simulink model "test_udp"  (R2021b)
settings: Solver=FixedStepAuto  StartTime=0.0  StopTime=inf  FixedStep=0.01  RelTol=1e-3
libraries: dspnetwork x3
settings Model: Creator=takeh  LastModifiedBy=takeh

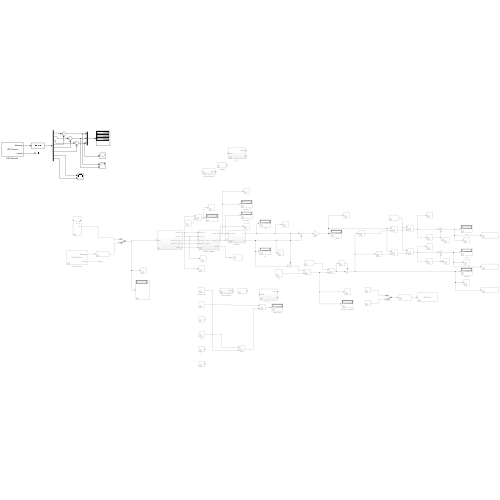
[thumbnail: Simulink's stored preview of the top-level diagram]
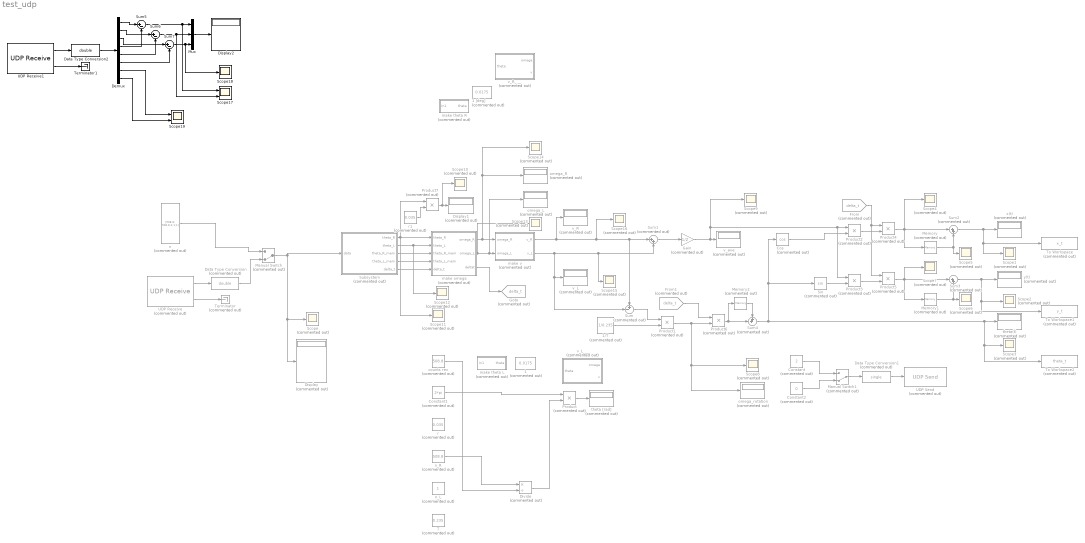
== system test_udp ==
  1 : Constant  Commented=on  Value=0.0175
  1 [deg] : Constant  Commented=on  Value=0.0175
  1/T : Constant  Commented=on  Value=1/0.235
  Constant : Constant  Commented=on  Value=2
  Constant1 : Constant  Commented=on  Value=2*pi
  Constant2 : Constant  Commented=on  Value=0
  Cos : Trigonometry  Commented=on  Operator=cos
  Data Type Conversion : DataTypeConversion  Commented=on  OutDataTypeStr=double
  Data Type Conversion1 : DataTypeConversion  Commented=on  OutDataTypeStr=single
  Data Type Conversion2 : DataTypeConversion  OutDataTypeStr=double
  Demux : Demux  Outputs=8
  Display : Display  Commented=on
  Display1 : Display  Commented=on
  Display2 : Display
  Divide : Product  Commented=on  Inputs=*/
  From : From  Commented=on  GotoTag=delta_t  TagVisibility=global
  From1 : From  Commented=on  GotoTag=delta_t  TagVisibility=global
  Gain : Gain  Commented=on  Gain=1/2
  Goto : Goto  Commented=on  GotoTag=delta_t  TagVisibility=global
  Manual Switch : ManualSwitch  Commented=on  CurrentSetting=0
  Manual Switch1 : ManualSwitch  Commented=on  CurrentSetting=0
  Memory : Memory  Commented=on
  Memory1 : Memory  Commented=on
  Memory2 : Memory  Commented=on
  Mux : Mux  Inputs=3
  Product{,1..7} (8 alike) : Product  Commented=on
  Scope{,1..16} (17 alike) : Scope  Commented=on
  Scope17 : Scope  NumInputPorts=2
  Scope18 : Scope
  Scope19 : Scope  NumInputPorts=2
  Sin : Trigonometry  Commented=on
  Subsystem : Subsystem  Commented=on
  Sum : Sum  Commented=on  Inputs=+-|
  Sum1 : Sum  Commented=on  Inputs=|++
  Sum2 : Sum  Commented=on  Inputs=|++
  Sum3 : Sum  Commented=on  Inputs=|++
  Sum4 : Sum  Commented=on  Inputs=++|
  Sum5 : Sum  Inputs=|+-
  Sum6 : Sum  Inputs=|+-
  Sum7 : Sum  Inputs=|+-
  T : Constant  Commented=on  Value=0.235
  Terminator : Terminator  Commented=on
  Terminator1 : Terminator
  To Workspace : ToWorkspace  Commented=on  VariableName=x_t  SaveFormat=Timeseries  SampleTime=-1
  To Workspace1 : ToWorkspace  Commented=on  VariableName=y_t  SaveFormat=Timeseries  SampleTime=-1
  To Workspace2 : ToWorkspace  Commented=on  VariableName=theta_t  SaveFormat=Timeseries  SampleTime=-1
  UDP Receive : dspnetwork/UDP Receive  Commented=on  localURL='0.0.0.0'  localPort=51000  remoteURL='127.0.0.1'  remotePort=-1  recvBufferSize=20  dims=5  signalDatatype=single  isComplex=off  isVarSize=off  showBlockingTime=off  blockingTime=0  sampletime=-1  blockPlatform=[]
  UDP Receive1 : dspnetwork/UDP Receive  localURL='0.0.0.0'  localPort=51000  remoteURL='127.0.0.1'  remotePort=-1  recvBufferSize=32  dims=8  signalDatatype=single  isComplex=off  isVarSize=off  showBlockingTime=off  blockingTime=0  sampletime=-1  blockPlatform=[]
  UDP Send : dspnetwork/UDP Send  Commented=on  remoteURL='127.0.0.1'  remotePort=52000  localURL='0.0.0.0'  localPortSource=Automatically determine  localPort=-1  sendBufferSize=8192  sampletime=-1  blockPlatform=[]  separateLengthPort=0
  counts rev : Constant  Commented=on  Value=508.8
  make omega : Subsystem  Commented=on
  make theta L : Subsystem  Commented=on
  make theta R : Subsystem  Commented=on
  make v : Subsystem  Commented=on
  n : Constant  Commented=on  Value=[508.8; 508.8;1;1;1]  VectorParams1D=off
  n_L : Constant  Commented=on
  n_R : Constant  Commented=on  Value=508.8
  omega_L : Display  Commented=on
  omega_R : Display  Commented=on
  omega_rotation : Display  Commented=on
  r : Constant  Commented=on  Value=0.035
  r1 : Constant  Commented=on  Value=0.035
  theta [rad] : Display  Commented=on
  theta(t) : Display  Commented=on
  v_L : Display  Commented=on
  v_L___ : Subsystem  Commented=on
  v_R : Display  Commented=on
  v_R____ : Subsystem  Commented=on
  v_ave : Display  Commented=on
  x(t) : Display  Commented=on
  y(t) : Display  Commented=on
  wires:
  UDP Receive/1 -> Data Type Conversion/1
  UDP Receive/2 -> Terminator/1
  Data Type Conversion/1 -> Manual Switch/2
  n/1 -> Manual Switch/1
  counts rev/1 -> Divide/2
  n_R/1 -> Divide/1
  Divide/1 -> Product/2
  Constant1/1 -> Product/1
  Product/1 -> theta [rad]/1
  1/T/1 -> Product1/2
  Sum/1 -> Product1/1
  Sum1/1 -> Gain/1
  Gain/1 -> Scope9/1, Product3/1, Product2/1, v_ave/1
  Sum4/1 -> To Workspace2/1, Scope3/1, theta(t)/1, Cos/1, Sin/1
  Cos/1 -> Product2/2
  Sin/1 -> Product3/2
  Sum3/1 -> y(t)/1, To Workspace1/1, Scope2/1
  make omega/1(omega_R) -> Scope14/1, omega_R/1, make v/1(omega_R)
  make v/1(v_R) -> Scope16/1, Sum1/1, Sum/1, v_R/1
  make v/2(v_L) -> Sum/2, v_L/1, Sum1/2, Scope15/1
  Constant/1 -> Manual Switch1/1
  Constant2/1 -> Manual Switch1/2
  Manual Switch1/1 -> Data Type Conversion1/1
  Data Type Conversion1/1 -> UDP Send/1
  Product2/1 -> Product4/2
  From/1 -> Product4/1, Product5/1
  Product3/1 -> Product5/2
  Sum2/1 -> x(t)/1, Scope1/1, To Workspace/1
  Memory/1 -> Sum2/2, Scope5/1
  Product5/1 -> Scope7/1, Memory1/1, Sum3/1
  Memory1/1 -> Scope6/1, Sum3/2
  Manual Switch/1 -> Subsystem/1(data), Scope/1, Display/1
  Subsystem/5(delta_t) -> make omega/5(delta_t)
  Subsystem/2(theta_L) -> Scope12/1, make omega/2(theta_L)
  Subsystem/3(theta_R_mem) -> make omega/3(theta_R_mem)
  Subsystem/4(theta_L_mem) -> make omega/4(theta_L_mem)
  make omega/3(deltat) -> Goto/1
  From1/1 -> Product6/1
  Product1/1 -> Product6/2, Scope8/1, omega_rotation/1
  Product6/1 -> Memory2/1, Sum4/2
  Memory2/1 -> Sum4/1
  Product4/1 -> Scope4/1, Sum2/1, Memory/1
  r1/1 -> Product7/2
  Product7/1 -> Scope10/1, Display1/1
  Subsystem/1(theta_R) -> Scope11/1, Product7/1, make omega/1(theta_R)
  make omega/2(omega_L) -> Scope13/1, make v/2(omega_L), omega_L/1
  UDP Receive1/1 -> Data Type Conversion2/1
  UDP Receive1/2 -> Terminator1/1
  Data Type Conversion2/1 -> Demux/1
  Demux/1 -> Sum5/1
  Demux/4 -> Sum5/2
  Demux/2 -> Sum6/1
  Demux/5 -> Sum6/2
  Demux/3 -> Sum7/1
  Demux/6 -> Sum7/2
  Sum6/1 -> Scope17/2, Mux/2
  Sum7/1 -> Scope18/1, Mux/3
  Sum5/1 -> Scope17/1, Mux/1
  Mux/1 -> Display2/1
  Demux/7 -> Scope19/1
  Demux/8 -> Scope19/2

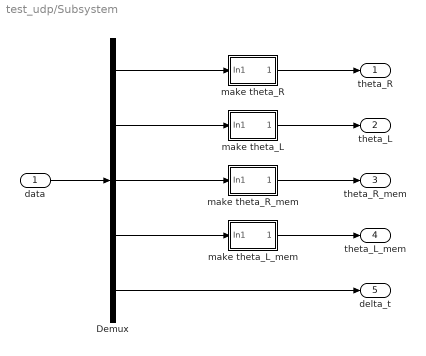
== system test_udp/Subsystem ==
  data : Inport
  Demux : Demux  Outputs=5
  make theta_L : Subsystem
  make theta_L_mem : Subsystem
  make theta_R : Subsystem
  make theta_R_mem : Subsystem
  theta_R : Outport
  theta_L : Outport  Port=2
  theta_R_mem : Outport  Port=3
  theta_L_mem : Outport  Port=4
  delta_t : Outport  Port=5
  wires:
  Demux/1 -> make theta_R/1(In1)
  make theta_R_mem/1(Out1) -> theta_R_mem/1
  Demux/3 -> make theta_R_mem/1(In1)
  make theta_L_mem/1(Out1) -> theta_L_mem/1
  Demux/2 -> make theta_L/1(In1)
  make theta_R/1(Out1) -> theta_R/1
  Demux/4 -> make theta_L_mem/1(In1)
  Demux/5 -> delta_t/1
  data/1 -> Demux/1
  make theta_L/1(Out1) -> theta_L/1

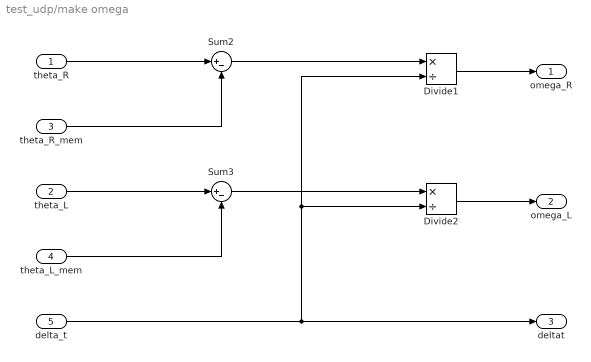
== system test_udp/make omega ==
  theta_R : Inport
  theta_L : Inport  Port=2
  theta_R_mem : Inport  Port=3
  theta_L_mem : Inport  Port=4
  delta_t : Inport  Port=5
  Divide1 : Product  Inputs=*/
  Divide2 : Product  Inputs=*/
  Sum2 : Sum  Inputs=|+-
  Sum3 : Sum  Inputs=|+-
  omega_R : Outport
  omega_L : Outport  Port=2
  deltat : Outport  Port=3
  wires:
  Sum2/1 -> Divide1/1
  Divide1/1 -> omega_R/1
  Sum3/1 -> Divide2/1
  Divide2/1 -> omega_L/1
  theta_R/1 -> Sum2/1
  theta_R_mem/1 -> Sum2/2
  theta_L/1 -> Sum3/1
  theta_L_mem/1 -> Sum3/2
  delta_t/1 -> deltat/1, Divide1/2, Divide2/2

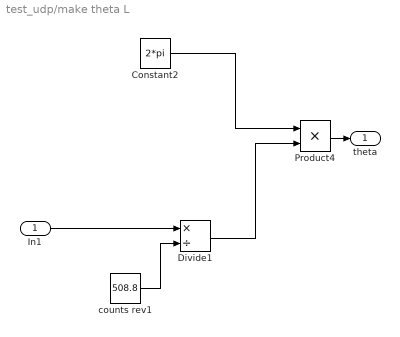
== system test_udp/make theta L ==
  In1 : Inport
  Constant2 : Constant  Value=2*pi
  Divide1 : Product  Inputs=*/
  Product4 : Product
  counts rev1 : Constant  Value=508.8
  theta : Outport
  wires:
  counts rev1/1 -> Divide1/2
  Constant2/1 -> Product4/1
  Divide1/1 -> Product4/2
  Product4/1 -> theta/1
  In1/1 -> Divide1/1

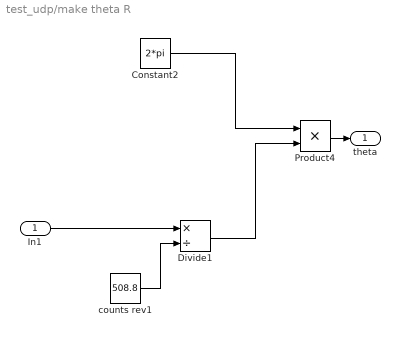
== system test_udp/make theta R ==
  In1 : Inport
  Constant2 : Constant  Value=2*pi
  Divide1 : Product  Inputs=*/
  Product4 : Product
  counts rev1 : Constant  Value=508.8
  theta : Outport
  wires:
  counts rev1/1 -> Divide1/2
  Constant2/1 -> Product4/1
  Divide1/1 -> Product4/2
  Product4/1 -> theta/1
  In1/1 -> Divide1/1

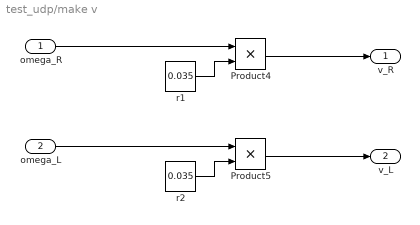
== system test_udp/make v ==
  omega_R : Inport
  omega_L : Inport  Port=2
  Product4 : Product
  Product5 : Product
  r1 : Constant  Value=0.035
  r2 : Constant  Value=0.035
  v_R : Outport
  v_L : Outport  Port=2
  wires:
  r2/1 -> Product5/2
  Product5/1 -> v_L/1
  Product4/1 -> v_R/1
  r1/1 -> Product4/2
  omega_R/1 -> Product4/1
  omega_L/1 -> Product5/1

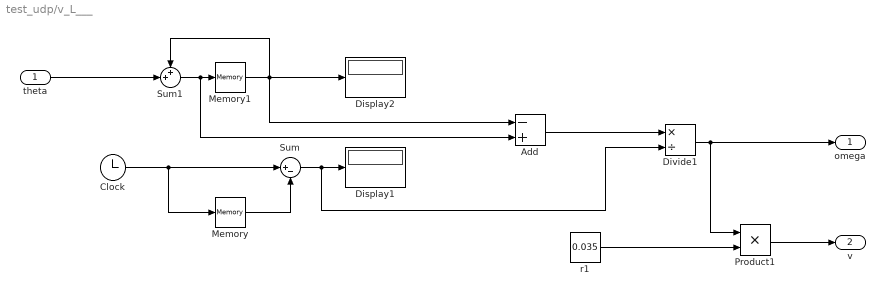
== system test_udp/v_L___ ==
  theta : Inport
  Add : Sum  Inputs=-+
  Clock : Clock
  Display1 : Display
  Display2 : Display
  Divide1 : Product  Inputs=*/
  Memory : Memory  InitialCondition=1
  Memory1 : Memory  InitialCondition=1
  Product1 : Product
  Sum : Sum  Inputs=|+-
  Sum1 : Sum  Inputs=++|
  r1 : Constant  Value=0.035
  omega : Outport
  v : Outport  Port=2
  wires:
  Memory1/1 -> Add/1, Display2/1, Sum1/1
  r1/1 -> Product1/2
  Sum1/1 -> Add/2, Memory1/1
  Sum/1 -> Divide1/2, Display1/1
  Memory/1 -> Sum/2
  Clock/1 -> Memory/1, Sum/1
  Add/1 -> Divide1/1
  Divide1/1 -> omega/1, Product1/1
  theta/1 -> Sum1/2
  Product1/1 -> v/1

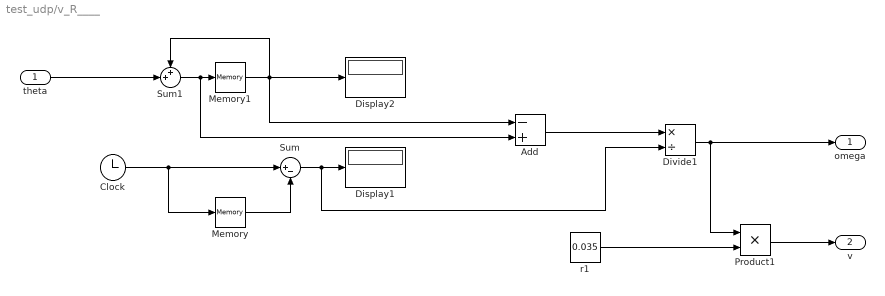
== system test_udp/v_R____ ==
  theta : Inport
  Add : Sum  Inputs=-+
  Clock : Clock
  Display1 : Display
  Display2 : Display
  Divide1 : Product  Inputs=*/
  Memory : Memory  InitialCondition=1
  Memory1 : Memory  InitialCondition=1
  Product1 : Product
  Sum : Sum  Inputs=|+-
  Sum1 : Sum  Inputs=++|
  r1 : Constant  Value=0.035
  omega : Outport
  v : Outport  Port=2
  wires:
  Memory1/1 -> Add/1, Display2/1, Sum1/1
  r1/1 -> Product1/2
  Sum1/1 -> Add/2, Memory1/1
  Sum/1 -> Divide1/2, Display1/1
  Memory/1 -> Sum/2
  Clock/1 -> Memory/1, Sum/1
  Add/1 -> Divide1/1
  Divide1/1 -> omega/1, Product1/1
  theta/1 -> Sum1/2
  Product1/1 -> v/1

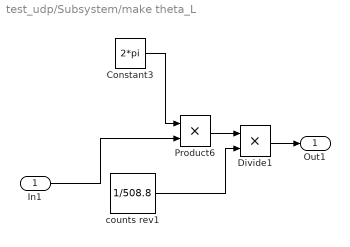
== system test_udp/Subsystem/make theta_L ==
  In1 : Inport
  Constant3 : Constant  Value=2*pi
  Divide1 : Product
  Product6 : Product
  counts rev1 : Constant  Value=1/508.8
  Out1 : Outport
  wires:
  Divide1/1 -> Out1/1
  In1/1 -> Product6/2
  counts rev1/1 -> Divide1/2
  Constant3/1 -> Product6/1
  Product6/1 -> Divide1/1

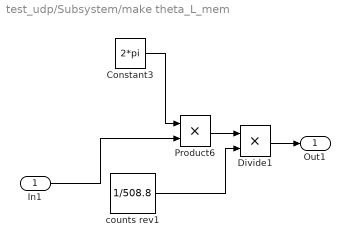
== system test_udp/Subsystem/make theta_L_mem ==
  In1 : Inport
  Constant3 : Constant  Value=2*pi
  Divide1 : Product
  Product6 : Product
  counts rev1 : Constant  Value=1/508.8
  Out1 : Outport
  wires:
  Divide1/1 -> Out1/1
  In1/1 -> Product6/2
  counts rev1/1 -> Divide1/2
  Constant3/1 -> Product6/1
  Product6/1 -> Divide1/1

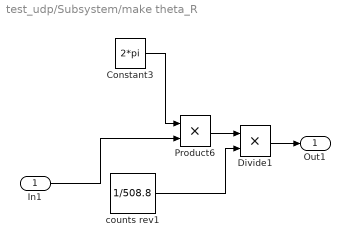
== system test_udp/Subsystem/make theta_R ==
  In1 : Inport
  Constant3 : Constant  Value=2*pi
  Divide1 : Product
  Product6 : Product
  counts rev1 : Constant  Value=1/508.8
  Out1 : Outport
  wires:
  Divide1/1 -> Out1/1
  In1/1 -> Product6/2
  counts rev1/1 -> Divide1/2
  Constant3/1 -> Product6/1
  Product6/1 -> Divide1/1

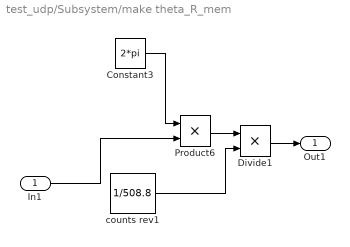
== system test_udp/Subsystem/make theta_R_mem ==
  In1 : Inport
  Constant3 : Constant  Value=2*pi
  Divide1 : Product
  Product6 : Product
  counts rev1 : Constant  Value=1/508.8
  Out1 : Outport
  wires:
  Divide1/1 -> Out1/1
  In1/1 -> Product6/2
  counts rev1/1 -> Divide1/2
  Constant3/1 -> Product6/1
  Product6/1 -> Divide1/1
